simulink model "fourbitlookaheadadder"  (R2017b)
settings: Solver=VariableStepAuto  StartTime=0.0  StopTime=10.0  RelTol=1e-3
libraries: hdlsllib x9
settings Model: Creator=Ray  LastModifiedBy=Ray

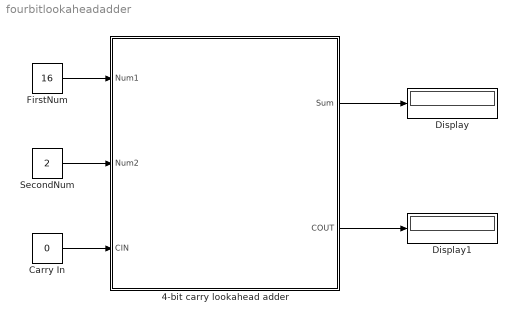
== system fourbitlookaheadadder ==
  4-bit carry lookahead adder : Subsystem
  Carry In : Constant  Value=0  OutDataTypeStr=boolean  SampleTime=1
  Display : Display
  Display1 : Display
  FirstNum : Constant  Value=16  OutDataTypeStr=uint8  SampleTime=1
  SecondNum : Constant  Value=2  OutDataTypeStr=uint8  SampleTime=1
  wires:
  FirstNum/1 -> 4-bit carry lookahead adder/1(Num1)
  SecondNum/1 -> 4-bit carry lookahead adder/2(Num2)
  Carry In/1 -> 4-bit carry lookahead adder/3(CIN)
  4-bit carry lookahead adder/1(Sum) -> Display/1
  4-bit carry lookahead adder/2(COUT) -> Display1/1

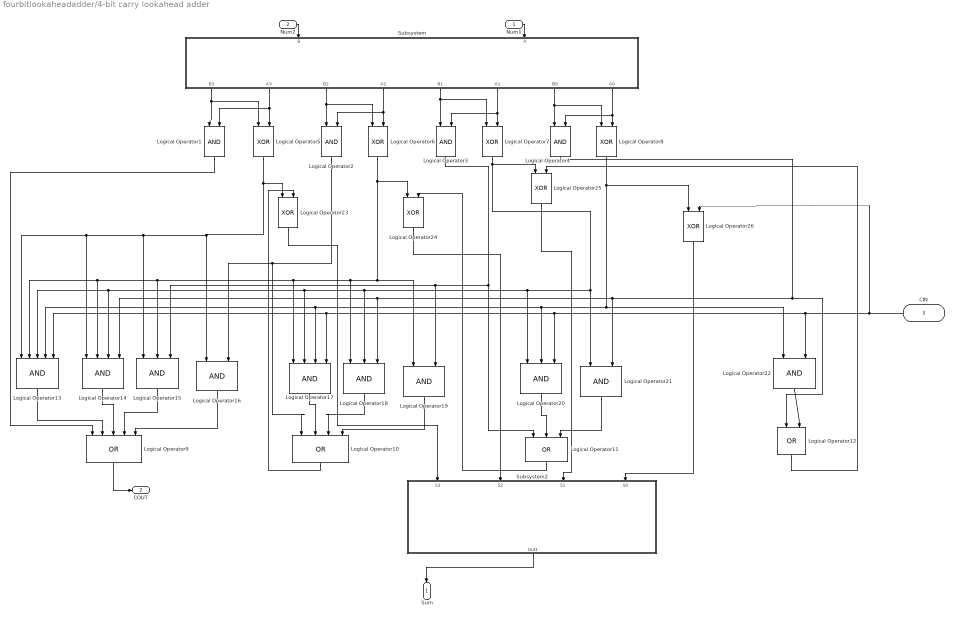
== system fourbitlookaheadadder/4-bit carry lookahead adder ==
  Num1 : Inport  SampleTime=1
  Num2 : Inport  Port=2  SampleTime=1
  CIN : Inport  Port=3  SampleTime=1
  Logical Operator{1..4,16,19,21..22} (8 alike) : Logic  IconShape=distinctive  AllPortsSameDT=off  OutDataTypeStr=boolean
  Logical Operator10 : Logic  Operator=OR  Inputs=4  IconShape=distinctive  AllPortsSameDT=off  OutDataTypeStr=boolean
  Logical Operator11 : Logic  Operator=OR  Inputs=3  IconShape=distinctive  AllPortsSameDT=off  OutDataTypeStr=boolean
  Logical Operator12 : Logic  Operator=OR  IconShape=distinctive  AllPortsSameDT=off  OutDataTypeStr=boolean
  Logical Operator13 : Logic  Inputs=5  IconShape=distinctive  AllPortsSameDT=off  OutDataTypeStr=boolean
  Logical Operator14 : Logic  Inputs=4  IconShape=distinctive  AllPortsSameDT=off  OutDataTypeStr=boolean
  Logical Operator15 : Logic  Inputs=3  IconShape=distinctive  AllPortsSameDT=off  OutDataTypeStr=boolean
  Logical Operator17 : Logic  Inputs=4  IconShape=distinctive  AllPortsSameDT=off  OutDataTypeStr=boolean
  Logical Operator18 : Logic  Inputs=3  IconShape=distinctive  AllPortsSameDT=off  OutDataTypeStr=boolean
  Logical Operator20 : Logic  Inputs=3  IconShape=distinctive  AllPortsSameDT=off  OutDataTypeStr=boolean
  Logical Operator{5..8,23..26} (8 alike) : Logic  Operator=XOR  IconShape=distinctive  AllPortsSameDT=off  OutDataTypeStr=boolean
  Logical Operator9 : Logic  Operator=OR  Inputs=5  IconShape=distinctive  AllPortsSameDT=off  OutDataTypeStr=boolean
  Subsystem : Subsystem
  Subsystem2 : Subsystem
  Sum : Outport  SampleTime=1
  COUT : Outport  Port=2  SampleTime=1
  wires:
  Logical Operator9/1 -> COUT/1
  Logical Operator19/1 -> Logical Operator10/4
  Subsystem2/1(Out1) -> Sum/1
  Logical Operator24/1 -> Subsystem2/2(S2)
  Logical Operator8/1 -> Logical Operator26/1, Logical Operator20/2, Logical Operator17/3, Logical Operator13/4, Logical Operator22/1
  Logical Operator4/1 -> Logical Operator21/2, Logical Operator18/3, Logical Operator14/4, Logical Operator12/1
  CIN/1 -> Logical Operator26/2, Logical Operator22/2, Logical Operator20/3, Logical Operator13/5, Logical Operator17/4
  Subsystem/7(B0) -> Logical Operator8/1, Logical Operator4/1
  Subsystem/2(A3) -> Logical Operator1/2, Logical Operator5/2
  Logical Operator22/1 -> Logical Operator12/2
  Logical Operator20/1 -> Logical Operator11/2
  Logical Operator17/1 -> Logical Operator10/2
  Subsystem/3(B2) -> Logical Operator6/1, Logical Operator2/1
  Logical Operator26/1 -> Subsystem2/4(S0)
  Logical Operator3/1 -> Logical Operator19/2, Logical Operator15/3, Logical Operator11/1
  Logical Operator2/1 -> Logical Operator10/1, Logical Operator16/2
  Logical Operator6/1 -> Logical Operator24/1, Logical Operator15/2, Logical Operator14/2, Logical Operator13/2, Logical Operator17/1, Logical Operator18/1, Logical Operator19/1
  Logical Operator21/1 -> Logical Operator11/3
  Num2/1 -> Subsystem/1(B)
  Logical Operator18/1 -> Logical Operator10/3
  Num1/1 -> Subsystem/2(A)
  Logical Operator7/1 -> Logical Operator25/1, Logical Operator20/1, Logical Operator18/2, Logical Operator17/2, Logical Operator14/3, Logical Operator13/3, Logical Operator21/1
  Logical Operator12/1 -> Logical Operator25/2
  Logical Operator5/1 -> Logical Operator23/1, Logical Operator15/1, Logical Operator14/1, Logical Operator13/1, Logical Operator16/1
  Logical Operator1/1 -> Logical Operator9/1
  Subsystem/5(B1) -> Logical Operator7/1, Logical Operator3/1
  Subsystem/1(B3) -> Logical Operator5/1, Logical Operator1/1
  Subsystem/4(A2) -> Logical Operator2/2, Logical Operator6/2
  Subsystem/8(A0) -> Logical Operator4/2, Logical Operator8/2
  Subsystem/6(A1) -> Logical Operator3/2, Logical Operator7/2
  Logical Operator23/1 -> Subsystem2/1(S3)
  Logical Operator15/1 -> Logical Operator9/4
  Logical Operator13/1 -> Logical Operator9/2
  Logical Operator14/1 -> Logical Operator9/3
  Logical Operator16/1 -> Logical Operator9/5
  Logical Operator10/1 -> Logical Operator23/2
  Logical Operator25/1 -> Subsystem2/3(S1)
  Logical Operator11/1 -> Logical Operator24/2

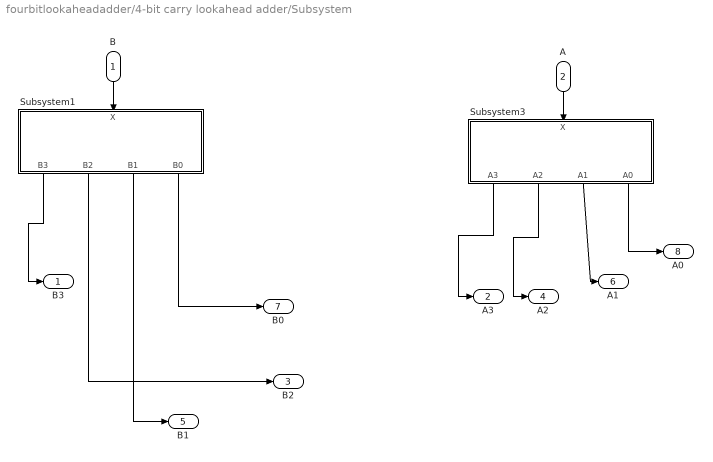
== system fourbitlookaheadadder/4-bit carry lookahead adder/Subsystem ==
  B : Inport
  A : Inport  Port=2
  Subsystem1 : Subsystem
  Subsystem3 : Subsystem
  B3 : Outport
  A3 : Outport  Port=2
  B2 : Outport  Port=3
  A2 : Outport  Port=4
  B1 : Outport  Port=5
  A1 : Outport  Port=6
  B0 : Outport  Port=7
  A0 : Outport  Port=8
  wires:
  Subsystem1/2(B2) -> B2/1
  Subsystem3/4(A0) -> A0/1
  Subsystem3/3(A1) -> A1/1
  Subsystem1/3(B1) -> B1/1
  Subsystem1/1(B3) -> B3/1
  Subsystem3/2(A2) -> A2/1
  Subsystem1/4(B0) -> B0/1
  Subsystem3/1(A3) -> A3/1
  A/1 -> Subsystem3/1(X)
  B/1 -> Subsystem1/1(X)

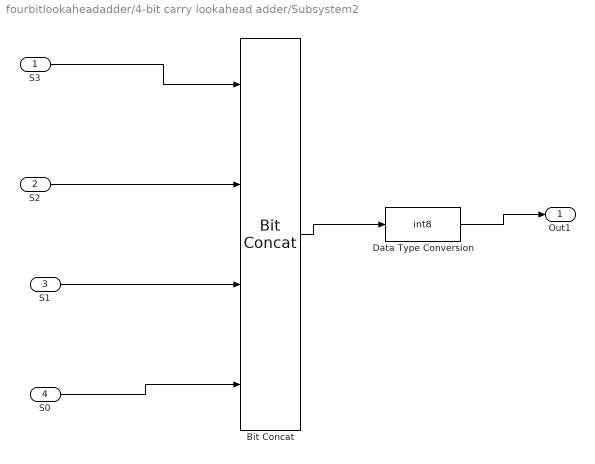
== system fourbitlookaheadadder/4-bit carry lookahead adder/Subsystem2 ==
  S3 : Inport
  S2 : Inport  Port=2
  S1 : Inport  Port=3
  S0 : Inport  Port=4
  Bit Concat : hdlsllib/Logic and Bit Operations/Bit Concat  numInputs=4
      settings: SourceProductName=HDL Coder  SourceProductBaseCode=HD
  Data Type Conversion : DataTypeConversion  OutDataTypeStr=int8
  Out1 : Outport
  wires:
  Bit Concat/1 -> Data Type Conversion/1
  Data Type Conversion/1 -> Out1/1
  S1/1 -> Bit Concat/3
  S2/1 -> Bit Concat/2
  S0/1 -> Bit Concat/4
  S3/1 -> Bit Concat/1

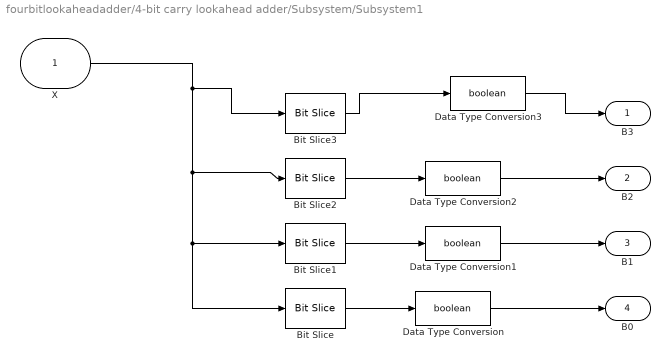
== system fourbitlookaheadadder/4-bit carry lookahead adder/Subsystem/Subsystem1 ==
  X : Inport  OutDataTypeStr=uint8  SampleTime=1
  Bit Slice : hdlsllib/Logic and Bit Operations/Bit Slice  lidx=0  ridx=0
  Bit Slice1 : hdlsllib/Logic and Bit Operations/Bit Slice  lidx=1  ridx=1
  Bit Slice2 : hdlsllib/Logic and Bit Operations/Bit Slice  lidx=2  ridx=2
  Bit Slice3 : hdlsllib/Logic and Bit Operations/Bit Slice  lidx=3  ridx=3
  Data Type Conversion{,1..3} (4 alike) : DataTypeConversion  OutDataTypeStr=boolean
  B3 : Outport
  B2 : Outport  Port=2
  B1 : Outport  Port=3
  B0 : Outport  Port=4
  wires:
  Data Type Conversion/1 -> B0/1
  Data Type Conversion1/1 -> B1/1
  X/1 -> Bit Slice/1, Bit Slice1/1, Bit Slice2/1, Bit Slice3/1
  Data Type Conversion3/1 -> B3/1
  Bit Slice2/1 -> Data Type Conversion2/1
  Bit Slice1/1 -> Data Type Conversion1/1
  Bit Slice/1 -> Data Type Conversion/1
  Data Type Conversion2/1 -> B2/1
  Bit Slice3/1 -> Data Type Conversion3/1

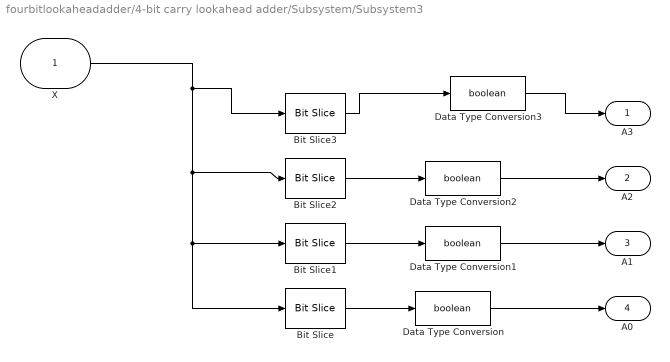
== system fourbitlookaheadadder/4-bit carry lookahead adder/Subsystem/Subsystem3 ==
  X : Inport  OutDataTypeStr=uint8  SampleTime=1
  Bit Slice : hdlsllib/Logic and Bit Operations/Bit Slice  lidx=0  ridx=0
  Bit Slice1 : hdlsllib/Logic and Bit Operations/Bit Slice  lidx=1  ridx=1
  Bit Slice2 : hdlsllib/Logic and Bit Operations/Bit Slice  lidx=2  ridx=2
  Bit Slice3 : hdlsllib/Logic and Bit Operations/Bit Slice  lidx=3  ridx=3
  Data Type Conversion{,1..3} (4 alike) : DataTypeConversion  OutDataTypeStr=boolean
  A3 : Outport
  A2 : Outport  Port=2
  A1 : Outport  Port=3
  A0 : Outport  Port=4
  wires:
  Data Type Conversion/1 -> A0/1
  Data Type Conversion1/1 -> A1/1
  X/1 -> Bit Slice/1, Bit Slice1/1, Bit Slice2/1, Bit Slice3/1
  Data Type Conversion3/1 -> A3/1
  Bit Slice2/1 -> Data Type Conversion2/1
  Bit Slice1/1 -> Data Type Conversion1/1
  Bit Slice/1 -> Data Type Conversion/1
  Data Type Conversion2/1 -> A2/1
  Bit Slice3/1 -> Data Type Conversion3/1
